simulink model "optimal_path_v1_3"  (R2019a)
settings: Solver=FixedStepDiscrete  StartTime=0.0  StopTime=inf  FixedStep=0.2  RelTol=1e-3  EnableMultiTasking=on
undefined symbols (not defined in the file): Data, Data_SL_Info
libraries: robotlib x17
settings Model: Creator=USER  LastModifiedBy=USER
settings SolverCC: InsertRTBMode=Never (minimum delay)
settings DataIOCC: ReturnWorkspaceOutputs=off
settings OptimizationCC: StrengthReduction=on  PassReuseOutputArgsAs=Individual arguments  MaxStackSize=64  OptimizeBlockOrder=speed  OptimizationPriority=Speed  OptimizationCustomize=off  MultiThreadedLoops=on
settings DebuggingCC: ParameterTunabilityLossMsg=error  PregeneratedLibrarySubsystemCodeDiagnostic=none  ArithmeticOperatorsInVariantConditions=warning
settings HardwareCC: ProdBitPerPointer=32  ProdBitPerSizeT=32  ProdBitPerPtrDiffT=32  ProdLargestAtomicFloat=None  ProdIntDivRoundTo=Undefined  ProdEndianess=Unspecified  ProdWordSize=32  ProdHWDeviceType=Generic->Unspecified (assume 32-bit Generic)
settings SFSimCC: SimUseLocalCustomCode=off  MATLABDynamicMemAlloc=off
settings RTWCC: SystemTargetFile=ert.tlc  HardwareBoard=Robot Operating System (ROS)  TLCOptions="-aInlineSetEventsForThisBaseRateFcn=TLC_FALSE -aSuppressMultiTaskScheduler=TLC_FALSE  -aRateBasedStepFcn=0"  TemplateMakefile=ert_default_tmf  GenerateReport=on  RTWUseLocalCustomCode=off  Toolchain=Catkin  BuildConfiguration=Faster Runs  IncludeHyperlinkInReport=on  LaunchReport=on  TargetLang=C++  GenerateTraceInfo=on  GenerateTraceReport=on  GenerateTraceReportSl=on  GenerateTraceReportSf=on  GenerateTraceReportEml=on
settings CodeAppCC: ForceParamTrailComments=on  IgnoreCustomStorageClasses=off  OperatorAnnotations=on  SimulinkDataObjDesc=on  SFDataObjDesc=on  InsertBlockDesc=on
settings ERTTargetCC: SupportVariableSizeSignals=on

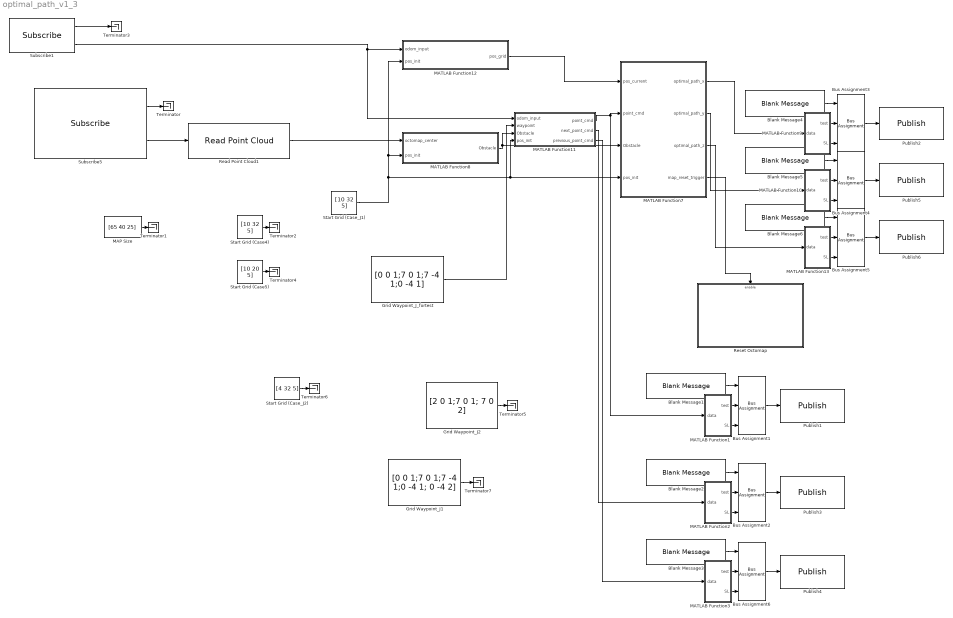
== system optimal_path_v1_3 ==
  Blank Message{1..6} (6 alike) : robotlib/Blank Message  messageClass=Message  entityType=std_msgs/Float32MultiArray  messageType=std_msgs/Float32MultiArray  SampleTime=-1
      settings: SourceProductBaseCode=RO
  Bus Assignment{1..6} (6 alike) : BusAssignment  AssignedSignals=Data,Data_SL_Info.CurrentLength
  Grid Waypoint_J1 : Constant  Value=[0 0 1;7 0 1;7 -4 1;0 -4 1; 0 -4 2]
  Grid Waypoint_J2 : Constant  Value=[2 0 1;7 0 1; 7 0 2]
  Grid Waypoint_J_fortest : Constant  Value=[0 0 1;7 0 1;7 -4 1;0 -4 1]
  MAP Size : Constant  Value=[65 40 25]
  MATLAB Function1 : MATLAB Function  TreatAsAtomicUnit=on
  MATLAB Function10 : MATLAB Function  TreatAsAtomicUnit=on
  MATLAB Function11 : MATLAB Function  TreatAsAtomicUnit=on
  MATLAB Function12 : MATLAB Function  TreatAsAtomicUnit=on
  MATLAB Function13 : MATLAB Function  TreatAsAtomicUnit=on
  MATLAB Function2 : MATLAB Function  TreatAsAtomicUnit=on
  MATLAB Function3 : MATLAB Function  TreatAsAtomicUnit=on
  MATLAB Function7 : MATLAB Function  TreatAsAtomicUnit=on
  MATLAB Function8 : MATLAB Function  TreatAsAtomicUnit=on
  MATLAB Function9 : MATLAB Function  TreatAsAtomicUnit=on
  Publish1 : robotlib/Publish  topicSource=Specify your own  topic=/current_point_cmd  messageType=std_msgs/Float32MultiArray  messageQueueLength=1
      settings: SourceProductBaseCode=RO
  Publish2 : robotlib/Publish  topicSource=Specify your own  topic=/optimal_path_x  messageType=std_msgs/Float32MultiArray  messageQueueLength=1
      settings: SourceProductBaseCode=RO
  Publish3 : robotlib/Publish  topicSource=Specify your own  topic=/next_point_cmd  messageType=std_msgs/Float32MultiArray  messageQueueLength=1
      settings: SourceProductBaseCode=RO
  Publish4 : robotlib/Publish  topicSource=Specify your own  topic=/previous_point_cmd  messageType=std_msgs/Float32MultiArray  messageQueueLength=1
      settings: SourceProductBaseCode=RO
  Publish5 : robotlib/Publish  topicSource=Specify your own  topic=/optimal_path_y  messageType=std_msgs/Float32MultiArray  messageQueueLength=1
      settings: SourceProductBaseCode=RO
  Publish6 : robotlib/Publish  topicSource=Specify your own  topic=/optimal_path_z  messageType=std_msgs/Float32MultiArray  messageQueueLength=1
      settings: SourceProductBaseCode=RO
  Read Point Cloud1 : robotlib/Read Point Cloud  MaximumPointCloudSize=[1, 650000]  PreserveStructure=off  ShowRGBOutput=off  ShowIntensityOutput=off  ShowErrorCodeOutput=off  VariableSizeOutputs=on
      settings: SourceProductName=Robotics System Toolbox  SourceProductBaseCode=RO
  "Reset Octomap " : Subsystem
  Start Grid (Case4) : Constant  Value=[10 32 5]
  Start Grid (Case5) : Constant  Value=[10 20 5]
  Start Grid (Case_J1) : Constant  Value=[10 32 5]
  Start Grid (Case_J2) : Constant  Value=[4 32 5]
  Subscribe1 : robotlib/Subscribe  topicSource=Select from ROS network  topic=/rtabmap/odom  messageType=nav_msgs/Odometry  sampleTime=-1  messageQueueLength=1
      settings: SourceProductBaseCode=RO
  Subscribe5 : robotlib/Subscribe  topicSource=Select from ROS network  topic=/octomap_point_cloud_centers  messageType=sensor_msgs/PointCloud2  sampleTime=-1  messageQueueLength=1
      settings: SourceProductBaseCode=RO
  Terminator{,1..7} (8 alike) : Terminator
  wires:
  MATLAB Function9/1(test) -> Bus Assignment3/2
  Blank Message4/1 -> Bus Assignment3/1
  Bus Assignment4/1 -> Publish5/1
  Blank Message5/1 -> Bus Assignment4/1
  MATLAB Function9/2(SL) -> Bus Assignment3/3
  Subscribe1/1 -> Terminator3/1
  Subscribe1/2 -> MATLAB Function11/1(odom_input), MATLAB Function12/1(odom_input)
  MATLAB Function13/2(SL) -> Bus Assignment5/3
  Start Grid (Case_J1)/1 -> MATLAB Function12/2(pos_init), MATLAB Function8/2(pos_init), MATLAB Function11/4(pos_init), MATLAB Function7/4(pos_init)
  MATLAB Function12/1(pos_grid) -> MATLAB Function7/1(pos_current)
  MATLAB Function10/1(test) -> Bus Assignment4/2
  MATLAB Function13/1(test) -> Bus Assignment5/2
  Bus Assignment5/1 -> Publish6/1
  MATLAB Function10/2(SL) -> Bus Assignment4/3
  Blank Message6/1 -> Bus Assignment5/1
  Bus Assignment3/1 -> Publish2/1
  MAP Size/1 -> Terminator1/1
  MATLAB Function8/1(Obstacle) -> MATLAB Function11/3(Obstacle), MATLAB Function7/3(Obstacle)
  MATLAB Function7/1(optimal_path_x) -> MATLAB Function9/1(data)
  MATLAB Function7/2(optimal_path_y) -> MATLAB Function10/1(data)
  MATLAB Function7/3(optimal_path_z) -> MATLAB Function13/1(data)
  Grid Waypoint_J_fortest/1 -> MATLAB Function11/2(waypoint)
  Read Point Cloud1/1 -> MATLAB Function8/1(octomap_center)
  Subscribe5/2 -> Read Point Cloud1/1
  Subscribe5/1 -> Terminator/1
  MATLAB Function7/4(map_reset_trigger) -> "Reset Octomap "/Enable
  Start Grid (Case4)/1 -> Terminator2/1
  Start Grid (Case5)/1 -> Terminator4/1
  Grid Waypoint_J2/1 -> Terminator5/1
  Start Grid (Case_J2)/1 -> Terminator6/1
  MATLAB Function1/2(SL) -> Bus Assignment1/3
  MATLAB Function1/1(test) -> Bus Assignment1/2
  MATLAB Function11/1(point_cmd) -> MATLAB Function1/1(data), MATLAB Function7/2(point_cmd)
  Blank Message1/1 -> Bus Assignment1/1
  Bus Assignment1/1 -> Publish1/1
  MATLAB Function2/2(SL) -> Bus Assignment2/3
  MATLAB Function2/1(test) -> Bus Assignment2/2
  MATLAB Function11/2(next_point_cmd) -> MATLAB Function2/1(data)
  Blank Message2/1 -> Bus Assignment2/1
  Bus Assignment2/1 -> Publish3/1
  Grid Waypoint_J1/1 -> Terminator7/1
  Blank Message3/1 -> Bus Assignment6/1
  MATLAB Function3/2(SL) -> Bus Assignment6/3
  MATLAB Function3/1(test) -> Bus Assignment6/2
  Bus Assignment6/1 -> Publish4/1
  MATLAB Function11/3(previous_point_cmd) -> MATLAB Function3/1(data)

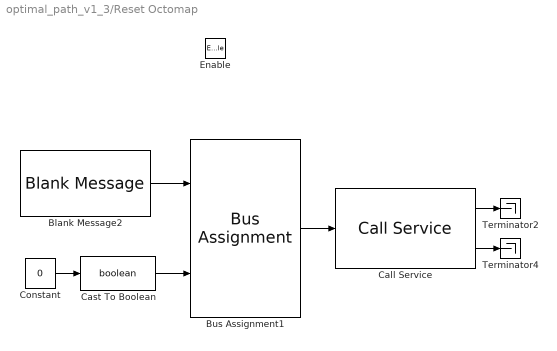
== system optimal_path_v1_3/Reset Octomap  ==
  Enable : EnablePort
  Blank Message2 : robotlib/Blank Message  messageClass=Service Request  entityType=std_srvs/Empty  messageType=std_srvs/EmptyRequest  SampleTime=inf
      settings: SourceProductBaseCode=RO
  Bus Assignment1 : BusAssignment  AssignedSignals=SL_DummyData
  Call Service : robotlib/Call Service  topicSource=Select from ROS network  service=/octomap_server/reset  serviceType=std_srvs/Empty  connectionTimeout=5  keepPersistent=off  ShowErrorCodeOutput=on
      settings: SourceProductName=Robotics System Toolbox  SourceProductBaseCode=RO
  Cast To Boolean : DataTypeConversion  OutDataTypeStr=boolean
  Constant : Constant  Value=0
  Terminator2 : Terminator
  Terminator4 : Terminator
  wires:
  Call Service/2 -> Terminator4/1
  Call Service/1 -> Terminator2/1
  Blank Message2/1 -> Bus Assignment1/1
  Bus Assignment1/1 -> Call Service/1
  Constant/1 -> Cast To Boolean/1
  Cast To Boolean/1 -> Bus Assignment1/2

== matlab function optimal_path_v1_3/MATLAB Function1 ==
  data: data input size=[1 3]; test output size=[1 128]; SL output
function [test,SL]   = func(data)

% test = single(nan(1,128));

test = single([data, nan(1,125)]);
% for i = 1:length(data)
%     test(i) = single(data(i));
% end

SL = uint32(length(data));


end

== matlab function optimal_path_v1_3/MATLAB Function2 ==
  data: data input size=[1 3]; test output size=[1 128]; SL output
function [test,SL]   = func(data)

% test = single(nan(1,128));

test = single([data, nan(1,125)]);
% for i = 1:length(data)
%     test(i) = single(data(i));
% end

SL = uint32(length(data));


end

== matlab function optimal_path_v1_3/MATLAB Function3 ==
  data: data input size=[1 3]; test output size=[1 128]; SL output
function [test,SL]   = func(data)

% test = single(nan(1,128));

test = single([data, nan(1,125)]);
% for i = 1:length(data)
%     test(i) = single(data(i));
% end

SL = uint32(length(data));


end

== matlab function optimal_path_v1_3/MATLAB Function10 ==
  data: data input size=[128 1]; test output size=[1 128]; SL output
function [test,SL]   = func(data)

% test = single(nan(1,128));

test = data';
% for i = 1:length(data)
%     test(i) = single(data(i));
% end

SL = uint32(length(data));


end

== matlab function optimal_path_v1_3/MATLAB Function11 ==
  data: odom_input input; waypoint input; point_cmd output; next_point_cmd output; previous_point_cmd output; Obstacle input; pos_init input
function [point_cmd, next_point_cmd,previous_point_cmd] = gen_waypoint(odom_input,waypoint,Obstacle,pos_init)

persistent waypoint_flag

if isempty(waypoint_flag)
    waypoint_flag = zeros(10,1);
end
grid_size=0.2;
% persistent flag
% 
% if isempty(flag)
%     flag = 1;
% end
% 
% pos_grid = int32(pos_grid);
% waypoint_x = waypoint(:,1);
% waypoint_y = waypoint(:,2);
% waypoint_z = waypoint(:,3);
% 
% point_cmd_test = int32([waypoint_x(flag) waypoint_y(flag) waypoint_z(flag)]);
% 
% if abs(point_cmd_test(1)-pos_grid(1)) <= 1 && abs(point_cmd_test(2)-pos_grid(2)) <= 1 && abs(point_cmd_test(3)-pos_grid(3)) <= 1
%     flag = flag + 1;
% end
% 
% if flag == numel(waypoint)/3 + 1
%     flag = numel(waypoint)/3;
% end
% 
% point_cmd = int32([waypoint_x(flag) waypoint_y(flag) waypoint_z(flag)]);

odom = zeros(1,3);
odom(1,1) = odom_input.Pose.Pose.Position.X;
odom(1,2) = odom_input.Pose.Pose.Position.Y;
odom(1,3) = odom_input.Pose.Pose.Position.Z;
waypoint_length = numel(waypoint)/3;

for a=1:waypoint_length
    % if Obstacle(int32(point_cmd/grid_size + pos_init'))==1
    if Obstacle(int32(waypoint(a,1)/grid_size + pos_init(1)),int32(waypoint(a,2)/grid_size + pos_init(2)),int32(waypoint(a,3)/grid_size + pos_init(3)))==1
        waypoint(a,:) = [waypoint(a,1)- cos(atan2(waypoint(a,2),waypoint(a,1))),waypoint(a,2)-sin(atan2(waypoint(a,2),waypoint(a,1))),waypoint(a,3)];
    end
end

waypoint_x = waypoint(:,1);
waypoint_y = waypoint(:,2);
waypoint_z = waypoint(:,3);
waypoint_path_norm = inf(waypoint_length,3);

waypoint_path_norm(:,1) = waypoint_x - odom(1);
waypoint_path_norm(:,2) = waypoint_y - odom(2);
waypoint_path_norm(:,3) = waypoint_z - odom(3);

K = inf(waypoint_length,1);

for i = 1:waypoint_length
    K(i) = norm(waypoint_path_norm(i,:));
end


% point_cmd = [odom(1,1) odom(1,2) odom(1,3)-10];  % Land (Maybe Hover)
if odom(1,3)<2.2
%     point_cmd = [odom(1,1) odom(1,2) odom(1,3)+0.2];
    point_cmd = [waypoint(end,1) waypoint(end,2) odom(1,3)+0.2];
else
    point_cmd = [odom(1,1) odom(1,2) odom(1,3)-10];  % Land (Maybe Hover) 
end
next_point_cmd = [-100,-3.5,1];  % 
previous_point_cmd = [0,0,0];  % 

% for j = 1:waypoint_length
%     if K(j) < 0.2
%         waypoint_flag(j) = 1;
%     end
% end

for i = 1:waypoint_length
    if waypoint_flag(i) == 0
        point_cmd = [waypoint_x(i), waypoint_y(i), waypoint_z(i)];
        if i < waypoint_length
            next_point_cmd = [waypoint_x(i+1), waypoint_y(i+1), waypoint_z(i+1)];
        else
            next_point_cmd = [waypoint_x(i)-waypoint_x(i-1), waypoint_y(i)-waypoint_y(i-1), waypoint_z(i)- waypoint_z(i-1)];
        end
        if i > 1
            previous_point_cmd = [waypoint_x(i-1), waypoint_y(i-1), waypoint_z(i-1)];
        end
        if K(i) < 0.2
            waypoint_flag(i) = 1;
        end
        
        break
    end
end


    
%     point_cmd = [waypoint_x(1) waypoint_y(1) waypoint_z(1)];
%     if K(1) < 0.2
%         waypoint_flag(1) = 1;
%     end
%     
%     if waypoint_flag(1) == 1
%         point_cmd = [waypoint_x(2) waypoint_y(2) waypoint_z(2)];
%     end
%     if K(2) < 0.2
%         waypoint_flag(2) = 1;
%     end
% 
% end
% if waypoint_flag(2) == 1
%     point_cmd = [waypoint_x(



% [~,m] = min(K);
% 
% if K(m) < 0.2
%     if m < waypoint_length
%         waypoint_flag(m) = 1;
%     end
% end
% 
% if waypoint_flag(m) == 1
%     point_cmd = [waypoint_x(m+1) waypoint_y(m+1) waypoint_z(m+1)];
% else
%     point_cmd = [waypoint_x(m) waypoint_y(m) waypoint_z(m)];
% end
% % waypoint_flag(m) = 1;
% 
% 
% 
% % [~,m] = min(K);
% % 
% % point_cmd = [waypoint_x(m) waypoint_y(m) waypoint_z(m)];

    

end

== matlab function optimal_path_v1_3/MATLAB Function12 ==
  data: odom_input input; pos_grid output; pos_init input
function pos_grid = odom_grid(odom_input,pos_init)

odom = zeros(1,3);


odom(1,1) = odom_input.Pose.Pose.Position.X;
odom(1,2) = odom_input.Pose.Pose.Position.Y;
odom(1,3) = odom_input.Pose.Pose.Position.Z;

start_point = [pos_init(1) pos_init(2) pos_init(3)];

% pos_x = int16(odom(1)/0.2+0.5);
% pos_y = int16(odom(2)/0.2+0.5);
% pos_z = int16(odom(3)/0.2+0.5);
pos_x = int16(odom(1)/0.2);
pos_y = int16(odom(2)/0.2);
pos_z = int16(odom(3)/0.2);

pos_grid = [pos_x+start_point(1) pos_y+start_point(2) pos_z+start_point(3)];


end

== matlab function optimal_path_v1_3/MATLAB Function13 ==
  data: data input size=[128 1]; test output size=[1 128]; SL output
function [test,SL]   = func(data)


% test = single(nan(1,128));

test = data';
% for i = 1:length(data)
%     test(i) = single(data(i));
% end

SL = uint32(length(data));

end

== matlab function optimal_path_v1_3/MATLAB Function7 ==
  data: pos_current input; optimal_path_x output size=[128 1]; point_cmd input; Obstacle input; pos_init input; optimal_path_y output size=[128 1]; optimal_path_z output size=[128 1]; map_reset_trigger output
function [optimal_path_x,optimal_path_y,optimal_path_z,map_reset_trigger] = Astar_algorithm_function(pos_current,point_cmd,Obstacle,pos_init)

persistent optimal sample hover_flag

if isempty(optimal)
    optimal = nan(128,3);
    hover_flag = 0;
    sample = 9;
end

% sample = sample + 1;
map_reset_trigger = 0;
grid_size = 0.2;

if Obstacle(pos_current(1), pos_current(2), pos_current(3)) ~= 1
    sample = sample + 1;
    if sample == 7
        map_reset_trigger = 1;
    end
end

if sample == 10
    sample = 1;
    
    mapsize = [65 40 25];
    
    
    Height = mapsize(1);        % x
    Width = mapsize(2);         % y
    Alt = mapsize(3);            % z
    
    Start = pos_current;
    Goal = int32(point_cmd/grid_size + pos_init');          % 수정
    look = 2;
    H_weight = 1.3;
    
    G_cost = zeros(2*look+1,2*look+1,2*look+1);
    for i = 1:2*look+1
        for j = 1:2*look+1
            for k = 1:2*look+1
                temp = [look+1 look+1 look+1]-[i j k];
                G_cost(i,j,k) = (min(sqrt(sum(abs(temp).^2,2))));
            end
        end
    end
    
    G_top2 = G_cost(:,:,1);
    G_top1 = G_cost(:,:,2);
    G_mid = G_cost(:,:,3);
    G_bottom1 = G_cost(:,:,4);
    G_bottom2 = G_cost(:,:,5);
    
    
    GScore = inf(Height,Width,Alt);
    GScore_temp = zeros(2*look+1,2*look+1,2*look+1);
    HScore = zeros(Height,Width,Alt);
    FScore = inf(Height,Width,Alt);
    ClosedMAT = zeros(Height,Width,Alt);
    CX = int32(Start(1));
    CY = int32(Start(2));
    CZ = int32(Start(3));
    ParentX = inf(Height,Width,Alt);
    ParentY = inf(Height,Width,Alt);
    ParentZ = inf(Height,Width,Alt);
    ParentX(CX,CY,CZ) = CX;
    ParentY(CX,CY,CZ) = CY;
    ParentZ(CX,CY,CZ) = CZ;
    hover_flag = 0;
    
    %%%%%%%%%%%%%%%% Define Heuristic %%%%%%%%%%%%%%%%%%%%%%%
    for k=1:Alt
        for j=1:Width
            for i=1:Height
                
                temp = (int32(Goal) - int32([i j k])) ;
                Distance=(min(sqrt(sum(abs(temp).^2,2))));
                HScore(i,j,k)=Distance*H_weight;               % (1+sqrt(2))/sqrt(3)
                
            end
        end
    end
    
    FScore(Start(1),Start(2),Start(3)) = HScore(Start(1),Start(2),Start(3));
    GScore(Start(1),Start(2),Start(3)) = 0;
    ClosedMAT(Obstacle==1)=1;
    REACHGOAL = 0;
    
    while 1
        
        MinFScore = min(min(min(FScore)));         % Find Minimun FScore
        
        if isinf(MinFScore)
            hover_flag = 1;
            break
        end
        
        
        [minF_x,minF_y] = find(FScore==MinFScore);
        HScore_temp = inf(1,10);
        
        minHScore = 1;
        for i = 1:length(minF_x)
            Current_pose_temp = [minF_x(i) rem(minF_y(i),Width) fix(minF_y(i)/Width)+1];     % H가 가장 적은걸로 먼저 선택
            CX_temp=Current_pose_temp(1);
            CY_temp=Current_pose_temp(2);
            CZ_temp=Current_pose_temp(3);
            HScore_temp(i) = HScore(CX_temp,CY_temp,CZ_temp);
            minHScore = find(HScore_temp == min(HScore_temp));
        end
        
        
        Current_pose = int32([minF_x(minHScore(1)) rem(minF_y(minHScore(1)),Width) fix(minF_y(minHScore(1))/Width)+1]);     % H가 가장 적은걸로 먼저 선택
        CX=Current_pose(1);
        CY=Current_pose(2);
        CZ=Current_pose(3);
        
        
        
        GScore_temp(:,:,1) = GScore(CX,CY,CZ) + G_top2;
        GScore_temp(:,:,2) = GScore(CX,CY,CZ) + G_top1;
        GScore_temp(:,:,3) = GScore(CX,CY,CZ) + G_mid;
        GScore_temp(:,:,4) = GScore(CX,CY,CZ) + G_bottom1;
        GScore_temp(:,:,5) = GScore(CX,CY,CZ) + G_bottom2;
        
        
        
        
        %%%%%%%%%%%%% GScore update %%%%%%%%%%%%%
        
        GScore(CX-look:CX+look,CY-look:CY+look,CZ+2) = min(GScore_temp(:,:,1),GScore(CX-look:CX+look,CY-look:CY+look,CZ+2)) ;
        GScore(CX-look:CX+look,CY-look:CY+look,CZ+1) = min(GScore_temp(:,:,2),GScore(CX-look:CX+look,CY-look:CY+look,CZ+1));
        GScore(CX-look:CX+look,CY-look:CY+look,CZ) = min(GScore_temp(:,:,3), GScore(CX-look:CX+look,CY-look:CY+look,CZ));
        GScore(CX-look:CX+look,CY-look:CY+look,CZ-1) = min(GScore_temp(:,:,4),GScore(CX-look:CX+look,CY-look:CY+look,CZ-1));
        GScore(CX-look:CX+look,CY-look:CY+look,CZ-2) = min(GScore_temp(:,:,5),GScore(CX-look:CX+look,CY-look:CY+look,CZ-2));
        
        
        FScore = GScore + HScore;
        %     ClosedMAT(CX,CY,CZ) = 1;
        ClosedMAT(CX-(look-1):CX+(look-1),CY-(look-1):CY+(look-1),CZ-(look-1):CZ+(look-1)) = 1;
        FScore(ClosedMAT==1) = inf;
        %     Check_FScore = FScore(CX-look:CX+look,CY-look:CY+look,CZ-look:CZ+look);
        
        
        
        [G_row1,G_col1] = find( GScore(CX-look:CX+look,CY-look:CY+look,CZ+2) == GScore_temp(:,:,1) );
        [G_row2,G_col2] = find( GScore(CX-look:CX+look,CY-look:CY+look,CZ+1) == GScore_temp(:,:,2) );
        [G_row3,G_col3] = find( GScore(CX-look:CX+look,CY-look:CY+look,CZ) == GScore_temp(:,:,3) );
        [G_row4,G_col4] = find( GScore(CX-look:CX+look,CY-look:CY+look,CZ-1) == GScore_temp(:,:,4) );
        [G_row5,G_col5] = find( GScore(CX-look:CX+look,CY-look:CY+look,CZ-2) == GScore_temp(:,:,5) );
        
        
        G_row1 = int32(G_row1);
        G_row2 = int32(G_row2);
        G_row3 = int32(G_row3);
        G_row4 = int32(G_row4);
        G_row5 = int32(G_row5);
        
        G_col1 = int32(G_col1);
        G_col2 = int32(G_col2);
        G_col3 = int32(G_col3);
        G_col4 = int32(G_col4);
        G_col5 = int32(G_col5);
        
        G_row1 = G_row1+CX-(look+1);
        G_row2 = G_row2+CX-(look+1);
        G_row3 = G_row3+CX-(look+1);
        G_row4 = G_row4+CX-(look+1);
        G_row5 = G_row5+CX-(look+1);
        
        G_col1 = G_col1+CY-(look+1);
        G_col2 = G_col2+CY-(look+1);
        G_col3 = G_col3+CY-(look+1);
        G_col4 = G_col4+CY-(look+1);
        G_col5 = G_col5+CY-(look+1);
        
        
        for i = 1:length(G_row1)
            ParentX(G_row1(i),G_col1(i),CZ+2) = CX;
            ParentY(G_row1(i),G_col1(i),CZ+2) = CY;
            ParentZ(G_row1(i),G_col1(i),CZ+2) = CZ;
        end
        
        for i = 1:length(G_row2)
            ParentX(G_row2(i),G_col2(i),CZ+1) = CX;
            ParentY(G_row2(i),G_col2(i),CZ+1) = CY;
            ParentZ(G_row2(i),G_col2(i),CZ+1) = CZ;
        end
        
        for i = 1:length(G_row3)
            if G_row3(i)==CX && G_col3(i)==CY
                continue
            end
            ParentX(G_row3(i),G_col3(i),CZ) = CX;
            ParentY(G_row3(i),G_col3(i),CZ) = CY;
            ParentZ(G_row3(i),G_col3(i),CZ) = CZ;
        end
        
        for i = 1:length(G_row4)
            ParentX(G_row4(i),G_col4(i),CZ-1) = CX;
            ParentY(G_row4(i),G_col4(i),CZ-1) = CY;
            ParentZ(G_row4(i),G_col4(i),CZ-1) = CZ;
        end
        
        for i = 1:length(G_row5)
            ParentX(G_row5(i),G_col5(i),CZ-2) = CX;
            ParentY(G_row5(i),G_col5(i),CZ-2) = CY;
            ParentZ(G_row5(i),G_col5(i),CZ-2) = CZ;
        end
        
        
        
        
        if abs(Goal(1)-CX)<=(look-1) && abs(Goal(2)-CY)<=(look-1) && abs(Goal(3)-CZ)<=(look-1)
            REACHGOAL = 1;
            break
        end
        
    end
    
    
    optimal = nan(128,3);
    if REACHGOAL
        optimal(1,:) = [Goal(1) Goal(2) Goal(3)];
        k=2;
        while 1
            CX_temp = int32(ParentX(CX,CY,CZ));
            CY_temp = int32(ParentY(CX,CY,CZ));
            CZ_temp = int32(ParentZ(CX,CY,CZ));
            
            CX = CX_temp;
            CY = CY_temp;
            CZ = CZ_temp;
            
            optimal(k,:) = [CX CY CZ];
            k = k+1;
            
            if CX==Start(1) && CY==Start(2) && CZ==Start(3)
                break
            end
        end
    end
    
end

% optimal_path_x = flip(single(((optimal(:,1)-pos_init(1))-0.5) * 0.2 + 0.1));      % grid_size = 0.2
% optimal_path_y = flip(single(((optimal(:,2)-pos_init(2))-0.5) * 0.2 + 0.1));
% optimal_path_z = flip(single(((optimal(:,3)-pos_init(3))-0.5) * 0.2 + 0.1));

if hover_flag == 1
    hover_point = nan(128,3);
    hover_point(1,:) = [pos_current(1) pos_current(2) pos_current(3)];
    optimal_path_x = flip(single( (hover_point(:,1)-pos_init(1)) * grid_size ));      % grid_size = 0.2,
    optimal_path_y = flip(single( (hover_point(:,2)-pos_init(2)) * grid_size ));
    optimal_path_z = flip(single( (hover_point(:,3)-pos_init(3)) * grid_size ));
else
    optimal_path_x = flip(single( (optimal(:,1)-pos_init(1)) * grid_size ));      % grid_size = 0.2
    optimal_path_y = flip(single( (optimal(:,2)-pos_init(2)) * grid_size ));
    optimal_path_z = flip(single( (optimal(:,3)-pos_init(3)) * grid_size ));
end

% if rmap_lost_flag == 1
%     optimal_path_x = single(nan(128,1));
%     optimal_path_y = single(nan(128,1));
%     optimal_path_z = single(nan(128,1));
% end


end

== matlab function optimal_path_v1_3/MATLAB Function8 ==
  data: octomap_center input size=[650000 3]; Obstacle output size=[65 40 25]; pos_init input
function Obstacle = gen_3d_array(octomap_center,pos_init)

mapsize = [65 40 25];

Obstacle = int8(zeros(mapsize(1),mapsize(2),mapsize(3)));
grid_size = 0.2;
start_point = [pos_init(1) pos_init(2) pos_init(3)];

% align1 = int16(octomap_center/(grid_size)+0.5);
align1 = int16(octomap_center/(grid_size));
align2 = unique(align1,'rows');
align3 = [align2(:,1)+start_point(1) align2(:,2)+start_point(2) align2(:,3)+start_point(3)];

for i = 1:numel(align3)/3
    
    index_temp = align3(i,:);
    
    index_check = index_temp<3;
    if sum(index_check)>=1
        index_temp(index_check) = 3;
    end
    
    if index_temp(1) > mapsize(1)-2
        index_temp(1) = mapsize(1)-2;
    end
    if index_temp(2) > mapsize(2)-2
        index_temp(2) = mapsize(2)-2;
    end
    if index_temp(3) > mapsize(3)-2
        index_temp(3) = mapsize(3)-2;
    end
    

    index_x = index_temp(1)-2:index_temp(1)+2;
    index_y = index_temp(2)-1:index_temp(2)+1;
    index_z = index_temp(3)-1:index_temp(3)+1;
%------------------------------------------------------------------------
%-----------------------------  scattering  -----------------------------
%------------------------------------------------------------------------
    Obstacle(index_x,index_temp(2)+1,index_temp(3)+1) = 1;
    Obstacle(index_x,index_temp(2)+1,index_temp(3)) = 1;
    Obstacle(index_x,index_temp(2)+1,index_temp(3)-1) = 1;
    Obstacle(index_x,index_temp(2),index_temp(3)+1) = 1;
    Obstacle(index_x,index_temp(2),index_temp(3)) = 1;
    Obstacle(index_x,index_temp(2),index_temp(3)-1) = 1;
    Obstacle(index_x,index_temp(2)-1,index_temp(3)+1) = 1;
    Obstacle(index_x,index_temp(2)-1,index_temp(3)) = 1;
    Obstacle(index_x,index_temp(2)-1,index_temp(3)-1) = 1;
    
    Obstacle(index_temp(1)+1,index_temp(2)+2,index_z) = 1;
    Obstacle(index_temp(1)+1,index_temp(2)-2,index_z) = 1;
    Obstacle(index_temp(1),index_temp(2)+2,index_z) = 1;
    Obstacle(index_temp(1),index_temp(2)-2,index_z) = 1;
    Obstacle(index_temp(1)-1,index_temp(2)+2,index_z) = 1;
    Obstacle(index_temp(1)-1,index_temp(2)-2,index_z) = 1;
    
    
    
    Obstacle(index_temp(1),index_y,index_temp(3)+2) = 1;
    Obstacle(index_temp(1),index_y,index_temp(3)-2) = 1;
    Obstacle(index_temp(1)+1,index_y,index_temp(3)+2) = 1;
    Obstacle(index_temp(1)+1,index_y,index_temp(3)-2) = 1;
    Obstacle(index_temp(1)-1,index_y,index_temp(3)+2) = 1;
    Obstacle(index_temp(1)-1,index_y,index_temp(3)-2) = 1;  %  Z FLAT Vehicle
    
    
    

%------------------------------------------------------------------------
%----------------------------  scattering 2  ----------------------------
%------------------------------------------------------------------------
    Obstacle(index_temp(1)+2,index_temp(2)+2,index_z) = 1;
    Obstacle(index_temp(1)+2,index_temp(2)+1,index_z) = 1;
    Obstacle(index_temp(1)+2,index_temp(2),index_z) = 1;
    Obstacle(index_temp(1)+2,index_temp(2)-1,index_z) = 1;
    Obstacle(index_temp(1)+2,index_temp(2)-2,index_z) = 1;
    
    Obstacle(index_temp(1)+1,index_temp(2)+2,index_z) = 1;
    Obstacle(index_temp(1)+1,index_temp(2)+1,index_z) = 1;
    Obstacle(index_temp(1)+1,index_temp(2),index_z) = 1;
    Obstacle(index_temp(1)+1,index_temp(2)-1,index_z) = 1;
    Obstacle(index_temp(1)+1,index_temp(2)-2,index_z) = 1;
    
    Obstacle(index_temp(1),index_temp(2)+2,index_z) = 1;
    Obstacle(index_temp(1),index_temp(2)+1,index_z) = 1;
    Obstacle(index_temp(1),index_temp(2),index_z) = 1;
    Obstacle(index_temp(1),index_temp(2)-1,index_z) = 1;
    Obstacle(index_temp(1),index_temp(2)-2,index_z) = 1;
    
    Obstacle(index_temp(1)-1,index_temp(2)+2,index_z) = 1;
    Obstacle(index_temp(1)-1,index_temp(2)+1,index_z) = 1;
    Obstacle(index_temp(1)-1,index_temp(2),index_z) = 1;
    Obstacle(index_temp(1)-1,index_temp(2)-1,index_z) = 1;
    Obstacle(index_temp(1)-1,index_temp(2)-2,index_z) = 1;
    
    Obstacle(index_temp(1)-2,index_temp(2)+2,index_z) = 1;
    Obstacle(index_temp(1)-2,index_temp(2)+1,index_z) = 1;
    Obstacle(index_temp(1)-2,index_temp(2),index_z) = 1;
    Obstacle(index_temp(1)-2,index_temp(2)-1,index_z) = 1;
    Obstacle(index_temp(1)-2,index_temp(2)-2,index_z) = 1;
    
end

Obstacle(1:3,:,:)=1;
Obstacle(mapsize(1)-2:mapsize(1),:,:) = 1;
Obstacle(:,1:3,:) = 1;
Obstacle(:,mapsize(2)-2:mapsize(2),:) = 1;
Obstacle(:,:,1:3) = 1;
% Obstacle(:,:,mapsize(3)-10:mapsize(3)) = 1; % 고도제한 2m 
Obstacle(:,:,mapsize(3)-8:mapsize(3)) = 1; % 고도제한 2.4m 

end

== matlab function optimal_path_v1_3/MATLAB Function9 ==
  data: data input size=[128 1]; test output size=[1 128]; SL output
function [test,SL]   = func(data)

% test = single(nan(1,128));

test = data';
% for i = 1:length(data)
%     test(i) = single(data(i));
% end

SL = uint32(length(data));


end
